simulink model "Knee_Joint"  (R2024b)
settings: Solver=VariableStepAuto  StartTime=0.0  StopTime=3  RelTol=1e-3
model workspace (MAT data in the model file):
  B = 0.001
  J = 0.0524
  Kb = 0.1146
  Kt = 0.1
  L = 0.0025
  R = 0.5
settings Model: Creator=reyes  LastModifiedBy=reyes
settings SolverCC: MaxConsecutiveMinStep=100

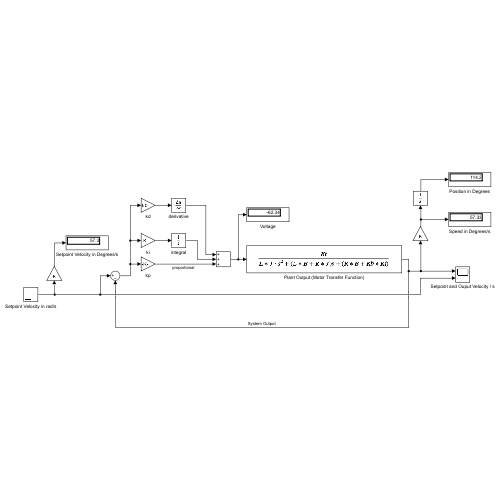
[thumbnail: Simulink's stored preview of the top-level diagram]
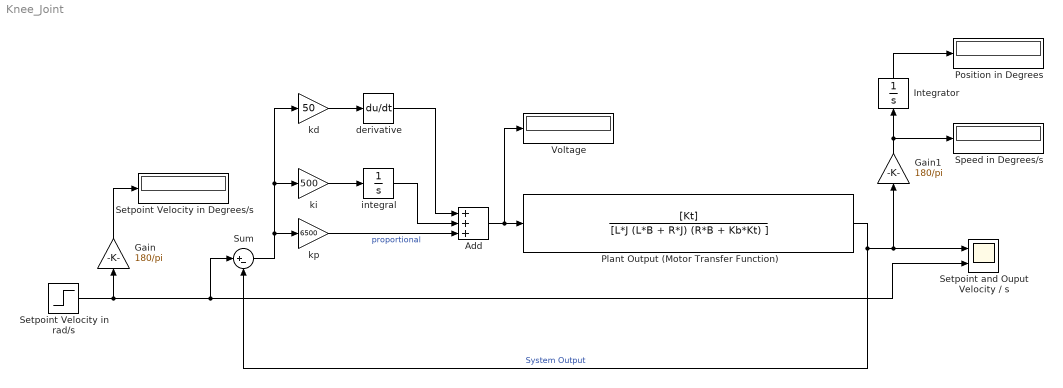
== system Knee_Joint ==
  Add : Sum  Inputs=+++
  Gain : Gain  Gain=180/pi
  Gain1 : Gain  Gain=180/pi
  Integrator : Integrator
  Plant Output (Motor Transfer Function) : TransferFcn  Numerator=[Kt]  Denominator=[L*J (L*B + R*J) (R*B + Kb*Kt) ]
  Position in Degrees : Display
  Setpoint Velocity in Degrees/s : Display
  Setpoint Velocity in rad/s : Step  SampleTime=0
  Setpoint and Ouput Velocity / s : Scope  NumInputPorts=2
  Speed in Degrees/s : Display
  Sum : Sum  Inputs=|+-
  Voltage : Display
  derivative : Derivative
  integral : Integrator
  kd : Gain  Gain=50
  ki : Gain  Gain=500
  kp : Gain  Gain=6500
  wires:
  Add/1 -> Voltage/1, Plant Output (Motor Transfer Function)/1
  Sum/1 -> kd/1, ki/1, kp/1
  kd/1 -> derivative/1
  ki/1 -> integral/1
  derivative/1 -> Add/1
  kp/1 -> Add/3  "proportional"
  integral/1 -> Add/2
  Plant Output (Motor Transfer Function)/1 -> Setpoint and Ouput Velocity / s/1, Gain1/1, Sum/2  "System Output"
  Setpoint Velocity in rad/s/1 -> Sum/1, Setpoint and Ouput Velocity / s/2, Gain/1
  Gain/1 -> Setpoint Velocity in Degrees/s/1
  Gain1/1 -> Integrator/1, Speed in Degrees/s/1
  Integrator/1 -> Position in Degrees/1
